simulink library "lib_GenTools_1DlinearInterp"  (R2015a)
settings: Solver=ode45  StartTime=0.0  StopTime=10.0  RelTol=1e-3
settings Model: Creator=jlkratz  LastModifiedBy=jlkratz

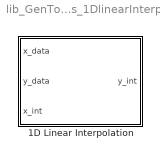
== system lib_GenTools_1DlinearInterp ==
  1D Linear Interpolation : Subsystem  mask(TSAT - 1D Linear Interpolation Block){BN_M=double(gcb)}
      mask prompts: BN_M "BN_M - Block Name"
      mask help: This block performs linear interpolation on a set of data (x_data, y_data) at interpolation points defined in the array x_int.
      mask Help: web(which('GenTools_TSAT_1DlinearInterp.html'),'-helpbrowser')

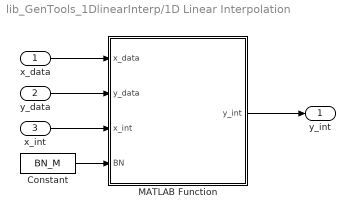
== system lib_GenTools_1DlinearInterp/1D Linear Interpolation ==
  x_data : Inport
  y_data : Inport  Port=2
  x_int : Inport  Port=3
  Constant : Constant  Value=BN_M
  MATLAB Function : MATLAB Function  TreatAsAtomicUnit=on
  y_int : Outport
  wires:
  x_data/1 -> MATLAB Function/1(x_data)
  Constant/1 -> MATLAB Function/4(BN)
  y_data/1 -> MATLAB Function/2(y_data)
  MATLAB Function/1(y_int) -> y_int/1
  x_int/1 -> MATLAB Function/3(x_int)

== matlab function lib_GenTools_1DlinearInterp/1D Linear Interpolation/MATLAB Function ==
  data: x_data input; y_int output; y_data input; x_int input; BN input
function y_int = interp1D(x_data,y_data,x_int,BN)
%#codegen

[n1,m1] = size(x_data);
[n2,m2] = size(y_data);
[n3,m3] = size(x_int);
diff_xdata = diff(x_data);

if min([n1,m1]) ~= 1
    y_int = ones(n3,m3);
    fprintf('Warning in %s: x_data must be a 1-D array. y_int has been set to an array of ones the size of x_int as a default.\n',char(BN));
elseif min([n2,m2]) ~= 1
    y_int = ones(n3,m3);
    fprintf('Warning in %s: y_data must be a 1-D array. y_int has been set to an array of ones the size of x_int as a default.\n',char(BN));
elseif min([n3,m3]) ~= 1
    y_int = ones(n3,m3);
    fprintf('Warning in %s: x_int must be a 1-D array. y_int has been set to an array of ones the size of x_int as a default.\n',char(BN));
elseif (n1 ~= n2) || (m1 ~= m2)
    y_int = ones(n3,m3);
    fprintf('Warning in %s: x_data and y_data must have the same dimensions. y_int has been set to an array of ones the size of x_int as a default.\n',char(BN));
elseif min(diff_xdata) <= 0
    y_int = ones(n3,m3);
    fprintf('Warning in %s: x_data must be monotonically increasing. y_int has been set to an array of ones the size of x_int as a default.\n',char(BN));
else
    y_int = zeros(n3,m3);
    for i = 1:length(x_int)
        if x_int(i) < x_data(1)
            y_int(i) = y_data(1);
            fprintf('Warning in %s: x_int(%-1.0i) is less than x_data(1). y_int(%-1.0i) has been set to y_data(1).\n',char(BN),int8(i),int8(i));
        elseif x_int(i) > x_data(end)
            y_int(i) = y_data(end);
            fprintf('Warning in %s: x_int(%-1.0i) is greater than x_data(end). y_int(%-1.0i) has been set to y_data(end).\n',char(BN),int8(i),int8(i));
        else
            y_int(i) = interp1(x_data,y_data,x_int(i));
        end
    end
end
